simulink model "ARCH_AT52_artificial"  (R2019b)
settings: Solver=FixedStepAuto  StartTime=0.0  StopTime=10.0  FixedStep=fixedStepSize  RelTol=1e-3
undefined symbols (not defined in the file): ARCH_AT52_timeHorizon, artificial_ARCH_AT5_constant, fixedStepSize
libraries: simulink x2
settings Model: Creator=JEDDELAN  LastModifiedBy=JEDDELAN
settings DataIOCC: SaveOutput=off  SaveTime=off  ReturnWorkspaceOutputs=off
settings DebuggingCC: ArithmeticOperatorsInVariantConditions=warning
settings SFSimCC: SimUseLocalCustomCode=off  CustomCodeUndefinedFunction=UseInterfaceOnly
settings RTWCC: RTWUseLocalCustomCode=off
settings GRTTargetCC: CombineOutputUpdateFcns=off  MatFileLogging=off

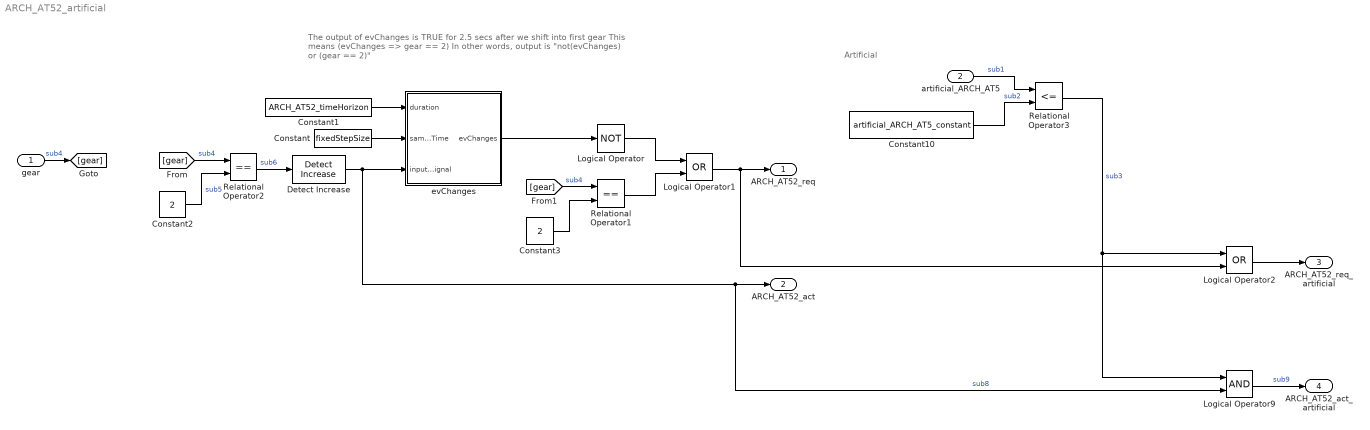
== system ARCH_AT52_artificial ==
  note: The output of evChanges is TRUE for 2.5 secs after we shift into first gear
      | This means (evChanges => gear == 2)
      | In other words, output is "not(evChanges) or (gear == 2)"
  note: Artificial
  gear : Inport
  artificial_ARCH_AT5 : Inport  Port=2
  Constant : Constant  Value=fixedStepSize
  Constant1 : Constant  Value=ARCH_AT52_timeHorizon
  Constant10 : Constant  Value=artificial_ARCH_AT5_constant
  Constant2 : Constant  Value=2
  Constant3 : Constant  Value=2
  Detect Increase : simulink/Logic and Bit Operations/Detect Increase  vinit=1  OutDataTypeStr=boolean
  Logical Operator : Logic  Operator=NOT  AllPortsSameDT=off  OutDataTypeStr=boolean
  Logical Operator1 : Logic  Operator=OR  AllPortsSameDT=off  OutDataTypeStr=boolean
  Logical Operator2 : Logic  Operator=OR  AllPortsSameDT=off  OutDataTypeStr=boolean
  Logical Operator9 : Logic  AllPortsSameDT=off  OutDataTypeStr=boolean
  Relational Operator1 : RelationalOperator  Operator===  OutDataTypeStr=boolean  RndMeth=Simplest
  Relational Operator2 : RelationalOperator  Operator===  OutDataTypeStr=boolean  RndMeth=Simplest
  Relational Operator3 : RelationalOperator  Operator=<=  OutDataTypeStr=boolean  RndMeth=Simplest
  evChanges : Subsystem
      settings: CopyFcn=set_param(gcbh,'LinkStatus','none');
  ARCH_AT52_req : Outport  OutDataTypeStr=boolean  PortDimensions=1  VectorParamsAs1DForOutWhenUnconnected=off
  ARCH_AT52_act : Outport  Port=2  OutDataTypeStr=boolean  PortDimensions=1  VectorParamsAs1DForOutWhenUnconnected=off
  ARCH_AT52_req_artificial : Outport  Port=3  OutDataTypeStr=boolean  PortDimensions=1  VectorParamsAs1DForOutWhenUnconnected=off
  ARCH_AT52_act_artificial : Outport  Port=4  OutDataTypeStr=boolean  PortDimensions=1  VectorParamsAs1DForOutWhenUnconnected=off
  wires:
  gear/1 -> [gear]  "sub4"
  Constant2/1 -> Relational Operator2/2  "sub5"
  Relational Operator2/1 -> Detect Increase/1  "sub6"
  evChanges/1(evChanges) -> Logical Operator/1
  Constant/1 -> evChanges/2(sampleTime)
  Constant1/1 -> evChanges/1(duration)
  [gear] -> Relational Operator2/1  "sub4"
  [gear] -> Relational Operator1/1  "sub4"
  Constant3/1 -> Relational Operator1/2
  Relational Operator1/1 -> Logical Operator1/2
  Logical Operator/1 -> Logical Operator1/1
  Constant10/1 -> Relational Operator3/2  "sub2"
  Logical Operator1/1 -> Logical Operator2/2, ARCH_AT52_req/1
  Relational Operator3/1 -> Logical Operator9/1, Logical Operator2/1  "sub3"
  Logical Operator2/1 -> ARCH_AT52_req_artificial/1
  artificial_ARCH_AT5/1 -> Relational Operator3/1  "sub1"
  Detect Increase/1 -> Logical Operator9/2, ARCH_AT52_act/1, evChanges/3(inputSignal)  "sub8"
  Logical Operator9/1 -> ARCH_AT52_act_artificial/1  "sub9"

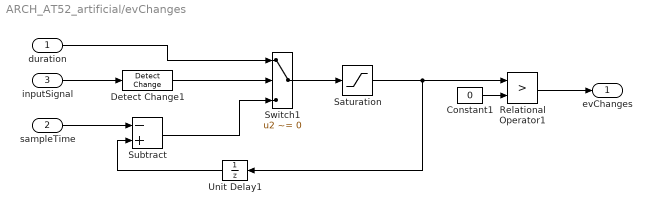
== system ARCH_AT52_artificial/evChanges ==
  duration : Inport
  sampleTime : Inport  Port=2
  inputSignal : Inport  Port=3
  Constant1 : Constant  Value=0
  Detect Change1 : simulink/Logic and Bit Operations/Detect Change  vinit=0  OutDataTypeStr=boolean
  Relational Operator1 : RelationalOperator  Operator=>  OutDataTypeStr=boolean  RndMeth=Nearest
  Saturation : Saturate  UpperLimit=Inf  LowerLimit=0
  Subtract : Sum  Inputs=-+
  Switch1 : Switch  Criteria=u2 ~= 0
  Unit Delay1 : UnitDelay  SampleTime=-1  HasFrameUpgradeWarning=on
  evChanges : Outport  VectorParamsAs1DForOutWhenUnconnected=off
  wires:
  Detect Change1/1 -> Switch1/2
  duration/1 -> Switch1/1
  Switch1/1 -> Saturation/1
  inputSignal/1 -> Detect Change1/1
  Constant1/1 -> Relational Operator1/2
  Subtract/1 -> Switch1/3
  Saturation/1 -> Relational Operator1/1, Unit Delay1/1
  Unit Delay1/1 -> Subtract/2
  Relational Operator1/1 -> evChanges/1
  sampleTime/1 -> Subtract/1
